simulink model "GTscalabilityModel"  (R2019b)
settings: Solver=VariableStepAuto  StartTime=0.0  StopTime=10.0  RelTol=1e-3
undefined symbols (not defined in the file): nb_rooms, nb_step_to_fifteen_min, nb_step_to_one_h, nb_step_to_thirty_min
libraries: dspstat3 x6
settings Model: Creator=pat  LastModifiedBy=pat

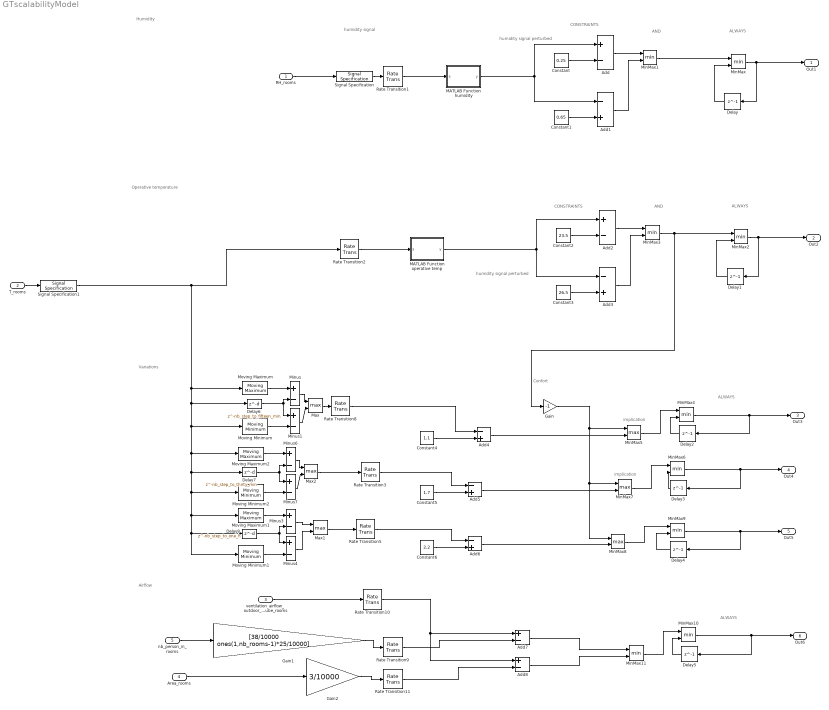
== system GTscalabilityModel ==
  note: implication
  note: Confort
  note: humidity signal perturbed
  note: CONSTRAINTS
  note: AND
  note: ALWAYS
  note: Humidity
  note: AND
  note: Operative temperature
  note: CONSTRAINTS
  note: ALWAYS
  note: ALWAYS
  note: Airflow
  note: Variations
  note: humidity signal
  note: humidity signal perturbed
  note: implication
  note: ALWAYS
  RH_rooms : Inport  PortDimensions=nb_rooms
  T_rooms : Inport  Port=2  PortDimensions=nb_rooms
  ventilation_airflow_outdoor_air_mcube_rooms : Inport  Port=3  PortDimensions=nb_rooms
  Area_rooms : Inport  Port=4  PortDimensions=nb_rooms
  nb_person_in_rooms : Inport  Port=5  OutDataTypeStr=double  PortDimensions=nb_rooms
  Add{,2,7..8} (4 alike) : Sum  Inputs=+-
  Add{1,3..6} (5 alike) : Sum  Inputs=-+
  Constant : Constant  Value=0.25
  Constant1 : Constant  Value=0.65
  Constant2 : Constant  Value=23.5
  Constant3 : Constant  Value=26.5
  Constant4 : Constant  Value=1.1
  Constant5 : Constant  Value=1.7
  Constant6 : Constant  Value=2.2
  Delay{,1..5} (6 alike) : Delay  DelayLength=1  InitialCondition=0
  Delay6 : Delay  DelayLength=nb_step_to_fifteen_min  InitialCondition=27
  Delay7 : Delay  DelayLength=nb_step_to_thirty_min  InitialCondition=27
  Delay8 : Delay  DelayLength=nb_step_to_one_h  InitialCondition=27
  Gain : Gain  Gain=-1
  Gain1 : Gain  Gain=[38/10000 ones(1,nb_rooms-1)*25/10000]
  Gain2 : Gain  Gain=3/10000
  MATLAB Function humidity : MATLAB Function  TreatAsAtomicUnit=on
  MATLAB Function operative temp : MATLAB Function  TreatAsAtomicUnit=on
  Max : MinMax  Function=max  Inputs=2  ZeroCross=off
  Max1 : MinMax  Function=max  Inputs=2  ZeroCross=off
  Max2 : MinMax  Function=max  Inputs=2  ZeroCross=off
  MinMax{,1..4,6,9..11} (9 alike) : MinMax  Inputs=2
  MinMax5 : MinMax  Function=max  Inputs=2
  MinMax7 : MinMax  Function=max  Inputs=2
  MinMax8 : MinMax  Function=max  Inputs=2
  Minus{,1,3..4,6..7} (6 alike) : Sum  Inputs=+-
  Moving Maximum : dspstat3/Moving Maximum  SpecifyWindowLength=on  WindowLength=nb_step_to_fifteen_min  SimulateUsing=Code generation
      settings: SourceProductName=DSP System Toolbox  SourceProductBaseCode=DS
  Moving Maximum1 : dspstat3/Moving Maximum  SpecifyWindowLength=on  WindowLength=nb_step_to_one_h  SimulateUsing=Code generation
      settings: SourceProductName=DSP System Toolbox  SourceProductBaseCode=DS
  Moving Maximum2 : dspstat3/Moving Maximum  SpecifyWindowLength=on  WindowLength=nb_step_to_thirty_min  SimulateUsing=Code generation
      settings: SourceProductName=DSP System Toolbox  SourceProductBaseCode=DS
  Moving Minimum : dspstat3/Moving Minimum  SpecifyWindowLength=on  WindowLength=nb_step_to_fifteen_min  SimulateUsing=Code generation
      settings: SourceProductName=DSP System Toolbox  SourceProductBaseCode=DS
  Moving Minimum1 : dspstat3/Moving Minimum  SpecifyWindowLength=on  WindowLength=nb_step_to_one_h  SimulateUsing=Code generation
      settings: SourceProductName=DSP System Toolbox  SourceProductBaseCode=DS
  Moving Minimum2 : dspstat3/Moving Minimum  SpecifyWindowLength=on  WindowLength=nb_step_to_thirty_min  SimulateUsing=Code generation
      settings: SourceProductName=DSP System Toolbox  SourceProductBaseCode=DS
  Rate Transition{1..3,5,8..11} (8 alike) : RateTransition  OutPortSampleTime=rate
  Signal Specification : SignalSpecification  OutMin=-0.25  OutMax=1.25  Dimensions=nb_rooms
  Signal Specification1 : SignalSpecification  OutMin=-100  OutMax=100  Dimensions=nb_rooms
  Out1 : Outport
  Out2 : Outport  Port=2
  Out3 : Outport  Port=3
  Out4 : Outport  Port=4
  Out5 : Outport  Port=5
  Out6 : Outport  Port=6
  wires:
  Delay/1 -> MinMax/2
  MinMax/1 -> Out1/1, Delay/1
  MinMax1/1 -> MinMax/1
  Delay1/1 -> MinMax2/2
  MinMax2/1 -> Out2/1, Delay1/1
  MATLAB Function humidity/1(y) -> Add/1, Add1/1
  Add/1 -> MinMax1/1
  Add1/1 -> MinMax1/2
  Constant/1 -> Add/2
  Constant1/1 -> Add1/2
  Add3/1 -> MinMax3/2
  Constant2/1 -> Add2/2
  Add2/1 -> MinMax3/1
  MATLAB Function operative temp/1(y) -> Add2/1, Add3/1
  Constant3/1 -> Add3/2
  Rate Transition1/1 -> MATLAB Function humidity/1(s)
  Rate Transition2/1 -> MATLAB Function operative temp/1(s)
  Delay2/1 -> MinMax4/2
  MinMax5/1 -> MinMax4/1
  MinMax4/1 -> Delay2/1, Out3/1
  MinMax3/1 -> Gain/1, MinMax2/1
  Add4/1 -> MinMax5/2
  Constant4/1 -> Add4/2
  Rate Transition8/1 -> Add4/1
  Gain/1 -> MinMax8/1, MinMax7/1, MinMax5/1
  MinMax6/1 -> Delay3/1, Out4/1
  MinMax7/1 -> MinMax6/1
  Delay3/1 -> MinMax6/2
  Add5/1 -> MinMax7/2
  Constant5/1 -> Add5/2
  Rate Transition3/1 -> Add5/1
  Constant6/1 -> Add6/2
  Rate Transition5/1 -> Add6/1
  Add6/1 -> MinMax8/2
  MinMax8/1 -> MinMax9/1
  MinMax9/1 -> Delay4/1, Out5/1
  Delay4/1 -> MinMax9/2
  Delay5/1 -> MinMax10/2
  MinMax10/1 -> Delay5/1, Out6/1
  MinMax11/1 -> MinMax10/1
  Rate Transition10/1 -> Add8/1, Add7/1
  Add7/1 -> MinMax11/1
  Rate Transition9/1 -> Add7/2
  Add8/1 -> MinMax11/2
  Rate Transition11/1 -> Add8/2
  Signal Specification/1 -> Rate Transition1/1
  RH_rooms/1 -> Signal Specification/1
  T_rooms/1 -> Signal Specification1/1
  Minus/1 -> Max/1
  Delay6/1 -> Minus1/1, Minus/2
  Minus1/1 -> Max/2
  Max/1 -> Rate Transition8/1
  Moving Minimum/1 -> Minus1/2
  Moving Maximum/1 -> Minus/1
  Moving Minimum2/1 -> Minus7/2
  Minus6/1 -> Max2/1
  Moving Maximum2/1 -> Minus6/1
  Delay7/1 -> Minus6/2, Minus7/1
  Minus7/1 -> Max2/2
  Max2/1 -> Rate Transition3/1
  Minus3/1 -> Max1/1
  Delay8/1 -> Minus3/2, Minus4/1
  Max1/1 -> Rate Transition5/1
  Minus4/1 -> Max1/2
  Moving Minimum1/1 -> Minus4/2
  Moving Maximum1/1 -> Minus3/1
  Signal Specification1/1 -> Moving Maximum/1, Moving Maximum2/1, Delay7/1, Moving Maximum1/1, Delay8/1, Moving Minimum1/1, Moving Minimum2/1, Moving Minimum/1, Delay6/1, Rate Transition2/1
  Gain2/1 -> Rate Transition11/1
  nb_person_in_rooms/1 -> Gain1/1
  Area_rooms/1 -> Gain2/1
  Gain1/1 -> Rate Transition9/1
  ventilation_airflow_outdoor_air_mcube_rooms/1 -> Rate Transition10/1

== matlab function GTscalabilityModel/MATLAB Function operative temp ==
  data: s input; y output
function y = fcn(s)
    function yy = fbis(ee)
        left = (s+ee)-23.5; 
        right = 26.5-(s+ee);    
        yy = min(left,right); % AND
    end

    [a b] =  fminbnd(@fbis,-1,1);  
    y=a;
end

== matlab function GTscalabilityModel/MATLAB Function humidity ==
  data: s input; y output
function y = fcn(s)
    function yy = fbis(ee)
        left = (s+ee)-0.25; 
        right = 0.65-(s+ee);    
        yy = min(left,right); % AND
    end

    [a b] =  fminbnd(@fbis,-1,1);  
    y=a;
end
